simulink model "example233s"  (R2017b)
settings: Solver=ode4  StartTime=0.0  StopTime=10.0  FixedStep=0.1  RelTol=1e-3
settings Model: Creator=GPL  LastModifiedBy=GPL

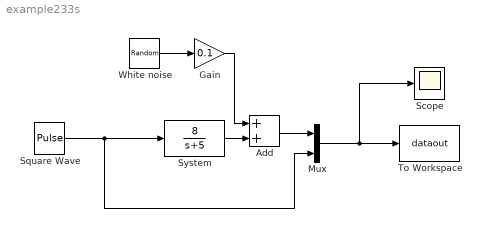
== system example233s ==
  Add : Sum
  Gain : Gain  Gain=0.1
  Mux : Mux  Inputs=2
  Scope : Scope
  Square Wave : DiscretePulseGenerator  PulseType=Time based  Period=5  PulseWidth=50
  System : TransferFcn  Numerator=[8]  Denominator=[1 5]  ContinuousStateAttributes='Plant'
  To Workspace : ToWorkspace  VariableName=dataout  SaveFormat=Timeseries  SampleTime=-1
  White noise : RandomNumber  Variance=0.1  SampleTime=0.1
  wires:
  Square Wave/1 -> Mux/2, System/1
  Mux/1 -> To Workspace/1, Scope/1
  Add/1 -> Mux/1
  System/1 -> Add/2
  White noise/1 -> Gain/1
  Gain/1 -> Add/1
